simulink model "Single_Quad"  (R2025b)
settings: Solver=ode4  StartTime=0.0  StopTime=80.0  FixedStep=0.001  RelTol=1e-3
values from neighbouring files (symbols this model uses):
  delta = zeros(3, 4)    [init_multi.m]    (also in init_single.m = [1; 1; 0]; plot_multi.m; plot_single.m = [1; 1; 0])
  g = 9.81    [init_multi.m]    (also in init_single.m)
  J = diag([0.04856, 0.04856, 0.08801])    [init_multi.m]    (also in init_single.m = diag([J_xx, J_yy, J_zz]))
  kp = 3    [init_multi.m]    (also in init_single.m)
  kt = 20    [init_multi.m]    (also in init_single.m)
  kv = 3    [init_multi.m]    (also in init_single.m)
  kw = 3    [init_multi.m]    (also in init_single.m)
  m = 1    [init_multi.m]    (also in init_single.m)
  p0 = [5; 3; -1]    [init_single.m]
  Q0 = [1; 0; 0; 0]    [init_single.m]
  v0 = [0; 0; 0]    [init_single.m]
  w0 = [0; 0; 0]    [init_single.m]
settings Model: Creator=ZhuanZ（无密码）  LastModifiedBy=ZhuanZ（无密码）
settings DataIOCC: ReturnWorkspaceOutputs=off

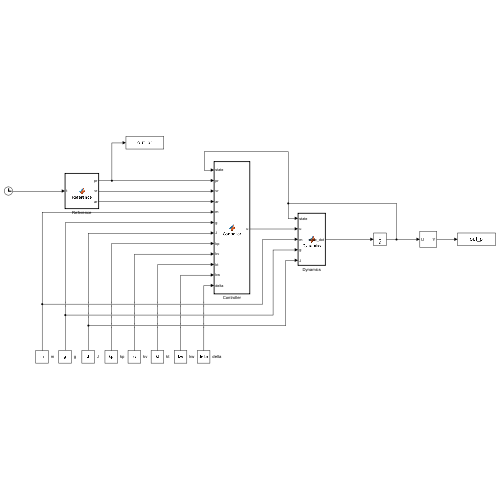
[thumbnail: Simulink's stored preview of the top-level diagram]
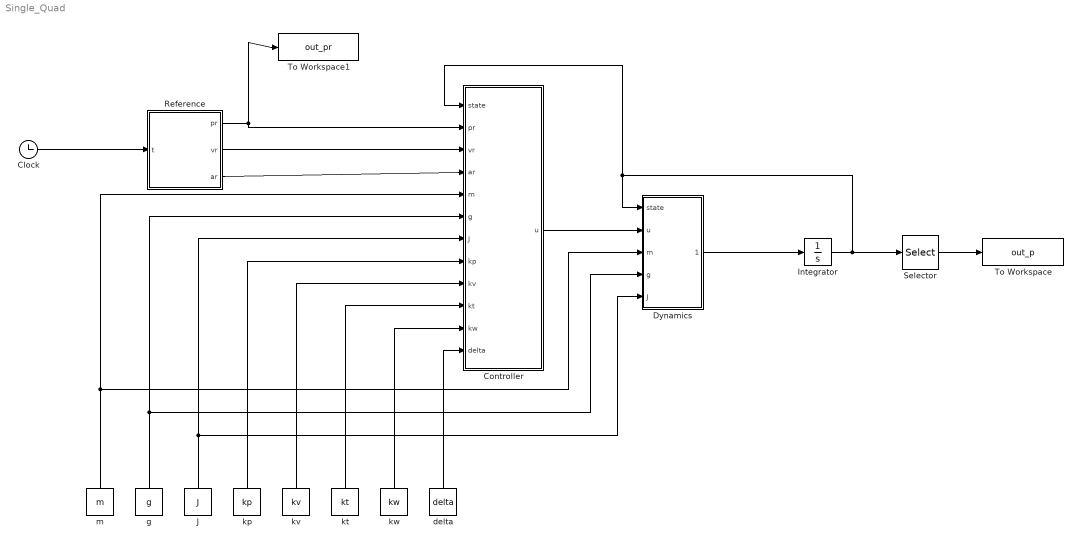
== system Single_Quad ==
  Clock : Clock
  Controller : MATLAB Function  TreatAsAtomicUnit=on
  Dynamics : MATLAB Function  TreatAsAtomicUnit=on
  Integrator : Integrator  InitialCondition=[p0; v0; Q0; w0]
  J : Constant  Value=J
  Reference : MATLAB Function  TreatAsAtomicUnit=on
  Selector : Selector  InputPortWidth=13  IndexOptions=Index vector (dialog)  Indices=[1 2 3]  OutputSizes=1
  To Workspace : ToWorkspace  VariableName=out_p  SaveFormat=Timeseries  SampleTime=-1
  To Workspace1 : ToWorkspace  VariableName=out_pr  SaveFormat=Timeseries  SampleTime=-1
  delta : Constant  Value=delta
  g : Constant  Value=g
  kp : Constant  Value=kp
  kt : Constant  Value=kt
  kv : Constant  Value=kv
  kw : Constant  Value=kw
  m : Constant  Value=m
  wires:
  Clock/1 -> Reference/1(t)
  Reference/3(ar) -> Controller/4(ar)
  Reference/2(vr) -> Controller/3(vr)
  Reference/1(pr) -> To Workspace1/1, Controller/2(pr)
  Controller/1(u) -> Dynamics/2(u)
  Dynamics/1(state_dot) -> Integrator/1
  Integrator/1 -> Dynamics/1(state), Controller/1(state), Selector/1
  m/1 -> Dynamics/3(m), Controller/5(m)
  g/1 -> Dynamics/4(g), Controller/6(g)
  J/1 -> Controller/7(J), Dynamics/5(J)
  kp/1 -> Controller/8(kp)
  kv/1 -> Controller/9(kv)
  kt/1 -> Controller/10(kt)
  kw/1 -> Controller/11(kw)
  delta/1 -> Controller/12(delta)
  Selector/1 -> To Workspace/1

== matlab function Single_Quad/Controller ==
  data: state input; u output; pr input; vr input; ar input; m input; g input; J input; kp input; kv input; kt input; kw input; delta input
function u = Controller(state, pr, vr, ar, m, g, J, kp, kv, kt, kw, delta)
    % 解包状态
    p = state(1:3);
    v = state(4:6);
    Q = state(7:10); % [sigma; q_vec]
    w = state(11:13);
    
    % --- 1. 位置环 (论文 Eq. 10) ---
    % 单机跟随模式：没有邻居，只跟领航者
    % 误差定义
    p_err = p - pr - delta;
    v_err = v - vr;
    
    e3 = [0;0;1];
    % 虚拟控制力 u_c
    % 注意：这里假设能直接获取 ar (完美观测器)，省去了复杂的 Estimator 模块
    u_c = m * (g*e3 + ar - kp * tanh(p_err) - kv * tanh(v_err));
    
    % --- 2. 姿态提取 (论文 Eq. 18 & Lemma 1) ---
    norm_uc = norm(u_c);
    if norm_uc < 1e-6
        norm_uc = 1e-6; % 防止分母为0
    end
    
    % 期望推力 T (Eq. 12)
    T = norm_uc;
    
    % 期望姿态 Qc = [sigma_c; qc_vec]
    u_z = u_c(3);
    % 论文 Eq. 18
    sigma_c = sqrt(0.5 * (1 + u_z/norm_uc));
    if sigma_c < 1e-6
        % 奇异点保护 (防止倒飞)
        sigma_c = 1e-6;
    end
    qc_vec = (1 / (2*norm_uc*sigma_c)) * [-u_c(2); u_c(1); 0];
    Qc = [sigma_c; qc_vec];
    
    % --- 3. 姿态环 (简化版) ---
    % 论文 Eq. 24 包含复杂的 wc_dot 前馈。
    % 为了新手复现成功，这里使用经典的四元数 PD 反馈，效果与论文几乎一致。
    
    % 计算姿态误差 Qe = Qc^{-1} * Q
    Qc_inv = [Qc(1); -Qc(2:4)];
    % 四元数乘法
    Qe_sigma = Qc_inv(1)*Q(1) - Qc_inv(2:4)'*Q(2:4);
    Qe_vec   = Qc_inv(1)*Q(2:4) + Q(1)*Qc_inv(2:4) + cross(Qc_inv(2:4), Q(2:4));
    
    % 保证最短路径 (若标量部小于0，取反)
    if Qe_sigma < 0
        Qe_vec = -Qe_vec;
    end
    
    % 力矩控制 (忽略陀螺力矩和前馈，只保留 PD)
    % we 近似为 w (假设目标角速度为0)
    tau = -kt * Qe_vec - kw * w;
    
    % 输出 [推力; 力矩x; 力矩y; 力矩z]
    u = [T; tau];
end

== matlab function Single_Quad/Reference ==
  data: t input; pr output; vr output; ar output
function [pr, vr, ar] = Reference(t)
    % 论文 Section IV 的 8 字形螺旋轨迹
    % pr: 位置, vr: 速度, ar: 加速度
    
    % 位置 pr = [3cos(0.2t), 2sin(0.2t), t]
    pr = [3*cos(0.2*t); 2*sin(0.2*t); t];
    
    % 速度 (对时间求导)
    vr = [-0.6*sin(0.2*t); 0.4*cos(0.2*t); 1];
    
    % 加速度 (再求导)
    ar = [-0.12*cos(0.2*t); -0.08*sin(0.2*t); 0];
end

== matlab function Single_Quad/Dynamics ==
  data: state input; u input; state_dot output; m input; g input; J input
function state_dot = Dynamics(state, u, m, g, J)
    % 解包
    p = state(1:3);
    v = state(4:6);
    Q = state(7:10); 
    w = state(11:13);
    
    T = u(1);     % 推力
    tau = u(2:4); % 力矩
    
    % 1. 位置导数
    p_dot = v;
    
    % 2. 速度导数 Eq. 3
    % R(Q) 计算
    s = Q(1); x = Q(2); y = Q(3); z = Q(4);
    R = [1-2*(y^2+z^2), 2*(x*y-s*z),   2*(x*z+s*y);
         2*(x*y+s*z),   1-2*(x^2+z^2), 2*(y*z-s*x);
         2*(x*z-s*y),   2*(y*z+s*x),   1-2*(x^2+y^2)];
     
    e3 = [0;0;1];
    v_dot = -g*e3 + (T/m) * R * e3;
    
    % 3. 四元数导数 Eq. 4
    % G(Q) * w * 0.5
    Q_dot = 0.5 * [ -x, -y, -z;
                     s, -z,  y;
                     z,  s, -x;
                    -y,  x,  s ] * w;
                
    % 4. 角速度导数 Eq. 5
    % J*w_dot = -cross(w, J*w) + tau
    w_dot = J \ (-cross(w, J*w) + tau);
    
    state_dot = [p_dot; v_dot; Q_dot; w_dot];
end
